simulink model "tqdtqr_rebuild_V3"  (R2021b)
settings: Solver=VariableStepAuto  StartTime=0.0  StopTime=10.0  RelTol=1e-3
undefined symbols (not defined in the file): ATQD_AfterTqMinGain_X_Deg, ATQD_APSCreepBaseTqD_X_kph, ATQD_APSCreepBaseTqD_Y_Deg, ATQD_APSCreepBaseTqR_X_kph, ATQD_APSCreepBaseTqR_Y_Deg, ATQD_APSCreepIterm_X_kph, ATQD_APSCreepIterm_Y_kph, ATQD_APSCreepPterm_X_kph, ATQD_APSCreepPterm_Y_kph, ATQD_APSDecReq_X_kph, ATQD_APSDecReq_Y_mps2, ATQD_APSDecReqCMD_X_kph, ATQD_APSDecReqTs_X_pct, ATQD_APSDecTimeGain_X_Deg, ATQD_APSDecTimeGain_Y_s, ATQD_APSReqLowSpd_X_Deg, ATQD_AutoHoldReleaseBPS_X_Deg, ATQD_AWDLoadTrqnsGain_X_kg, ATQD_AWDLoadTrqnsGain_Y_pct, ATQD_BOSEnBPSPosn_X_kph, ATQD_BOSMap_X_rpm, ATQD_BOSMap_Y_pct, ATQD_CreepBaseTqD_X_kph, ATQD_CreepBaseTqD_Y_Deg, ATQD_CreepBaseTqR_X_kph, ATQD_CreepBaseTqR_Y_Deg, ATQD_CreepBPSDisPosn_X_Deg, ATQD_CreepBPSDisPosnR_X_Deg, ATQD_CreepBPSEnPosn_X_Deg, ATQD_CreepBPSEnPosnR_X_Deg, ATQD_CreepDeltaTq_X_kph, ATQD_CreepIterm_X_kph, ATQD_CreepIterm_Y_kph, ATQD_CreepItermMaxLimit_X_pct, ATQD_CreepPreloadTime_X_kph, ATQD_CreepPreloadTq_X_kph, ATQD_CreepPreloadTq_Y_s, ATQD_CreepProtTq_X_Deg, ATQD_CreepPterm_X_kph, ATQD_CreepPterm_Y_kph, ATQD_CreepRrTqSpRat_X_rpm, ATQD_CreepRrTqSpRat_Y_Nm, ATQD_CreepTargetSpdD_X_pct, ATQD_CreepTargetSpdR_X_pct, ATQD_CreepUpLimitTq_X_rpm, ATQD_DecIneOPDHoldEnDelay_X_Deg, ATQD_DecIneOPDHoldEnDelay_Y_bar, ATQD_ECOTqMapD_X_rpm, ATQD_ECOTqMapD_Y_pct, ATQD_EMTqMapD_X_rpm, ATQD_EMTqMapD_Y_pct, ATQD_EOPDTqMapDCon_X_rpm, ATQD_EOPDTqMapDCon_Y_Deg, ATQD_EstInitVehWeight_X_c, ATQD_FAfterTqCMDGain_X_rpm, ATQD_FAfterTqCMDGain_Y_pct, ATQD_ForceLowSpd_X_Deg, ATQD_ForcePLimitSpd_X_Deg, ATQD_FrLossMAPLowV_X_rpm, ATQD_FrLossMAPLowV_Y_Nm ... (+949)
libraries: simulink x235, hcu_lib x208, tqr x63, tqd x6
(part 19 of 37)

== system tqdtqr_rebuild_V3/Input_Convert/Main function/Front//Rear ramp parameters determine/Front First order filter input tau map and determination ==
  note: Drive mode case
  note: Determine Tq by different case
  VTQD_TqTargetShaftSpd_rpm : Inport
  VTQR_EVDriveMode_enum : Inport  Port=2
  VTQD_RollRegenEnable_flg : Inport  Port=3
  VTQD_TqSourceFr_enum : Inport  Port=4
  VTQR_FEDUWhlTqReqSmoothDelay_Nm : Inport  Port=5
  VDHP_ActAPSPosn_pct : Inport  Port=6
  VINP_VehSpeed_kph : Inport  Port=7
  VTQD_LimpHomeAct_flg : Inport  Port=8
  VTQD_EVDriveModeValid_flg : Inport  Port=9
  VTQD_RegenMode_enum : Inport  Port=10
  VVMC_ACCPedalOvrd_flg : Inport  Port=11
  VVMC_CCPedalOvrd_flg : Inport  Port=12
  VTQD_PreLoadHold_flg : Inport  Port=13
  VVMC_ActMaxSlideRate_pct : Inport  Port=14
  VTQD_CreepPrLoadEnable_flg : Inport  Port=15
  VTQD_RDCActive_enum : Inport  Port=16
  VTQR_NoABSFEDUWhlTqReq_Nm : Inport  Port=17
  VTQR_RampFEDUWhlTqReq_Nm : Inport  Port=18
  VTQR_FrFirstOrderInpTq_Nm : Inport  Port=19
  VTQD_PedAccTqEn_flg : Inport  Port=20
  VTQD_PreLoadPreEn_flg : Inport  Port=21
  VVMC_MSAWhlTqActive_flg : Inport  Port=22
  VINP_FrPTCSActive_flg : Inport  Port=23
  VINP_IVISnowModeCmd_flg : Inport  Port=24
  VTQD_IVIRockModeEn_flg : Inport  Port=25
  VINP_VehicleType_enum : Inport  Port=26
  VTQD_CoordWhlTqDemFr_Nm : Inport  Port=27
  VINP_FrntAxlTrqReqDrv_Nm : Inport  Port=28
  VVMC_EstSlope_Deg : Inport  Port=29
  AND : Logic  AllPortsSameDT=off  OutDataTypeStr=boolean
  AND1 : Logic  Inputs=3  AllPortsSameDT=off  OutDataTypeStr=boolean
  AND2 : Logic  Inputs=3  AllPortsSameDT=off  OutDataTypeStr=boolean
  AND3 : Logic  AllPortsSameDT=off  OutDataTypeStr=boolean
  AND4 : Logic  AllPortsSameDT=off  OutDataTypeStr=boolean
  Abs : Abs
  Abs4 : Abs
  Add : Sum  Inputs=+-
  Add1 : Sum  Inputs=+-
  Constant : Constant  Value=ENUM_VEHICLETYPE_D31L24
  Constant1 : Constant  Value=ENUM_TQSOURCE_APS
  Constant10 : Constant  Value=KTQR_PreLoadTs_c
  Constant11 : Constant  Value=ENUM_DRIVEMODE_ECO
  Constant12 : Constant  Value=ENUM_DRIVEMODE_NRM
  Constant16 : Constant  Value=ENUM_DRIVEMODE_SPORT
  Constant2 : Constant  Value=KTQR_DriveModeCMDTqDev_Nm
  Constant3 : Constant  Value=ENUM_TQSOURCE_CC
  Constant32 : Constant  Value=KTQR_TIPOutTsAPS_pct
  Constant33 : Constant  Value=KTQR_TIPOutTsSpd_kph
  Constant34 : Constant  Value=ENUM_TQSOURCE_ADAS
  Constant5 : Constant  Value=KTQR_ARegenLatchEnTq_Nm
  Constant6 : Constant  Value=KTQR_PreLoadPreEnTs_c
  Constant7 : Constant  Value=ENUM_RDCACTSTA_NOREQUEST
  Constant8 : Constant  Value=KTQR_DriveModeChangeTq_Nm
  Constant9 : Constant  Value=ENUM_TQSOURCE_MSA
  Creep : Subsystem  TreatAsAtomicUnit=on
  Delay : Delay  DelayLength=1
  Delay1 : Delay  DelayLength=1
  Delay2 : Delay  DelayLength=1
  Detect Change : simulink/Logic and Bit Operations/Detect Change  vinit=0  OutDataTypeStr=boolean
  Drive mode : Subsystem  TreatAsAtomicUnit=on
  Equal : RelationalOperator  Operator=~=  OutDataTypeStr=boolean  RndMeth=Simplest
  Equal10 : RelationalOperator  Operator===  OutDataTypeStr=boolean  RndMeth=Simplest
  Equal11 : RelationalOperator  Operator===  OutDataTypeStr=boolean  RndMeth=Simplest
  Equal2 : RelationalOperator  Operator=~=  OutDataTypeStr=boolean  RndMeth=Simplest
  Equal9 : RelationalOperator  Operator===  OutDataTypeStr=boolean  RndMeth=Simplest
  GreaterThan2 : RelationalOperator  OutDataTypeStr=boolean  RndMeth=Simplest
  If : If  NumInputs=7  IfExpression=u1~= 0  ElseIfExpressions=u2 ~= 0, u3 ~= 0,u4~=0,u5~=0,u6~=0
  If1 : If  NumInputs=6  IfExpression=u1~= 0  ElseIfExpressions=u2 ~= 0, u3 ~= 0,u4~=0,u5~=0,u6~=0
  Less Than2 : RelationalOperator  Operator=<=  OutDataTypeStr=boolean  RndMeth=Simplest
  Logical Operator : Logic  AllPortsSameDT=off  OutDataTypeStr=boolean
  Logical Operator1 : Logic  Inputs=3  AllPortsSameDT=off  OutDataTypeStr=boolean
  Logical Operator14 : Logic  Operator=OR  Inputs=5  AllPortsSameDT=off  OutDataTypeStr=boolean
  Logical Operator2 : Logic  Operator=OR  AllPortsSameDT=off  OutDataTypeStr=boolean
  Logical Operator3 : Logic  Operator=NOT  AllPortsSameDT=off  OutDataTypeStr=boolean
  Logical Operator4 : Logic  Operator=NOT  AllPortsSameDT=off  OutDataTypeStr=boolean
  Logical Operator5 : Logic  AllPortsSameDT=off  OutDataTypeStr=boolean
  Merge : Merge  Inputs=7
  Merge1 : Merge  Inputs=7
  NOT : Logic  Operator=NOT  AllPortsSameDT=off  OutDataTypeStr=boolean
  NOT1 : Logic  Operator=NOT  AllPortsSameDT=off  OutDataTypeStr=boolean
  OR2 : Logic  Operator=OR  AllPortsSameDT=off  OutDataTypeStr=boolean
  Preleoad : Subsystem  TreatAsAtomicUnit=on
  PreleoadPreEn : Subsystem  TreatAsAtomicUnit=on
  RDCActive : Subsystem  TreatAsAtomicUnit=on
  Relational Operator : RelationalOperator  Operator=>  OutDataTypeStr=boolean  RndMeth=Simplest
  Relational Operator1 : RelationalOperator  Operator=~=  OutDataTypeStr=boolean  RndMeth=Simplest
  Relational Operator2 : RelationalOperator  Operator=<=  OutDataTypeStr=boolean  RndMeth=Simplest
  Relational Operator3 : RelationalOperator  Operator===  OutDataTypeStr=boolean  RndMeth=Simplest
  Relational Operator4 : RelationalOperator  Operator===  OutDataTypeStr=boolean  RndMeth=Simplest
  Relational Operator5 : RelationalOperator  Operator=<  OutDataTypeStr=boolean  RndMeth=Simplest
  Relational Operator6 : RelationalOperator  OutDataTypeStr=boolean  RndMeth=Simplest
  Relational Operator7 : RelationalOperator  Operator===  OutDataTypeStr=boolean  RndMeth=Simplest
  SR_Latch1 : hcu_lib/Basic_Blocks/SR_Latch
  Switch4 : Switch  Criteria=u2 > Threshold
  TIP : Subsystem  TreatAsAtomicUnit=on
  VMC : Subsystem  TreatAsAtomicUnit=on
  VTQR_ECOFEDUTs_c : tqr/TQR/Determine Torque Request/TorqueArbitrament/TorqueSmooth/Front First order filter input tau map and determination/VTQR_ECOFEDUTs_c  SystemSampleTime=-1  VariantActivationTime=update diagram  Latency=0  AutoFrameSizeCalculation=off
  VTQR_ESCAPEFEDUTs_c : tqr/TQR/Determine Torque Request/TorqueArbitrament/TorqueSmooth/Front First order filter input tau map and determination/VTQR_ESCAPEFEDUTs_c  SystemSampleTime=-1  VariantActivationTime=update diagram  Latency=0  AutoFrameSizeCalculation=off
  VTQR_LHMFEDUTs_c : tqr/TQR/Determine Torque Request/TorqueArbitrament/TorqueSmooth/Front First order filter input tau map and determination/VTQR_LHMFEDUTs_c  SystemSampleTime=-1  VariantActivationTime=update diagram  Latency=0  AutoFrameSizeCalculation=off
  VTQR_NORMALFEDUTs_c : tqr/TQR/Determine Torque Request/TorqueArbitrament/TorqueSmooth/Front First order filter input tau map and determination/VTQR_NORMALFEDUTs_c  SystemSampleTime=-1  VariantActivationTime=update diagram  Latency=0  AutoFrameSizeCalculation=off
  VTQR_SNOWFEDUTs_c : tqr/TQR/Determine Torque Request/TorqueArbitrament/TorqueSmooth/Front First order filter input tau map and determination/VTQR_SNOWFEDUTs_c  SystemSampleTime=-1  VariantActivationTime=update diagram  Latency=0  AutoFrameSizeCalculation=off
  VTQR_SPORTFEDUTs_c : tqr/TQR/Determine Torque Request/TorqueArbitrament/TorqueSmooth/Front First order filter input tau map and determination/VTQR_SPORTFEDUTs_c  SystemSampleTime=-1  VariantActivationTime=update diagram  Latency=0  AutoFrameSizeCalculation=off
  VTQR_TCSFEDUTs_c : tqr/TQR/Determine Torque Request/TorqueArbitrament/TorqueSmooth/Front First order filter input tau map and determination/VTQR_TCSFEDUTs_c  SystemSampleTime=-1  VariantActivationTime=update diagram  Latency=0  AutoFrameSizeCalculation=off
  VTQR_FrFirstOrderInpTs_c : Outport
  wires:
  VTQD_CoordWhlTqDemFr_Nm/1 -> [VTQD_CoordWhlTqDemFr_Nm]
  VINP_FrntAxlTrqReqDrv_Nm/1 -> [VINP_FrntAxlTrqReqDrv_Nm]
  VINP_VehicleType_enum/1 -> [VINP_VehicleType_enum]
  VINP_IVISnowModeCmd_flg/1 -> [VINP_IVISnowModeCmd_flg]
  VTQD_IVIRockModeEn_flg/1 -> [VTQD_IVIRockModeEn_flg]
  VINP_FrPTCSActive_flg/1 -> [VINP_FrPTCSActive_flg]
  [VTQD_PedAccTqEn_flg] -> Logical Operator14/5
  AND3/1 -> Logical Operator14/3
  Constant9/1 -> Relational Operator7/2
  [VVMC_MSAWhlTqActive_flg] -> AND3/2
  VVMC_MSAWhlTqActive_flg/1 -> [VVMC_MSAWhlTqActive_flg]
  [VTQD_TqSourceFr_enum] -> Relational Operator7/1
  Relational Operator7/1 -> AND3/1
  VTQD_PreLoadPreEn_flg/1 -> [VTQD_PreLoadPreEn_flg]
  VTQD_PedAccTqEn_flg/1 -> [VTQD_PedAccTqEn_flg]
  VVMC_ActMaxSlideRate_pct/1 -> [VVMC_ActMaxSlideRate_pct]
  VTQR_FrFirstOrderInpTq_Nm/1 -> [VTQR_FrFirstOrderInpTq_Nm]
  [VTQR_RampFEDUWhlTqReq_Nm] -> Relational Operator2/1
  Constant7/1 -> Equal2/2
  Equal2/1 -> AND/2
  [VTQD_RDCActive_enum] -> Equal2/1
  Relational Operator2/1 -> AND/1
  Constant5/1 -> Relational Operator2/2
  VTQR_RampFEDUWhlTqReq_Nm/1 -> [VTQR_RampFEDUWhlTqReq_Nm]
  VTQR_NoABSFEDUWhlTqReq_Nm/1 -> [VTQR_NoABSFEDUWhlTqReq_Nm]
  VTQD_RDCActive_enum/1 -> [VTQD_RDCActive_enum]
  VTQD_CreepPrLoadEnable_flg/1 -> [VTQD_CreepPrLoadEnable_flg]
  VTQD_PreLoadHold_flg/1 -> [VTQD_PreLoadHold_flg]
  VVMC_CCPedalOvrd_flg/1 -> [VVMC_CCPedalOvrd_flg]
  VVMC_ACCPedalOvrd_flg/1 -> [VVMC_ACCPedalOvrd_flg]
  GreaterThan2/1 -> AND2/2
  [VTQD_TqSourceFr_enum] -> Relational Operator4/1
  Relational Operator1/1 -> AND2/3
  Relational Operator3/1 -> Logical Operator14/1
  Logical Operator14/1 -> AND1/1
  Constant33/1 -> GreaterThan2/2
  Constant3/1 -> Relational Operator3/2
  Less Than2/1 -> AND2/1
  [VTQD_TqSourceFr_enum] -> Relational Operator3/1
  [VDHP_ActAPSPosn_pct] -> Less Than2/1
  Relational Operator4/1 -> Logical Operator14/2
  Constant32/1 -> Less Than2/2
  Constant34/1 -> Relational Operator4/2
  [VINP_VehSpeed_kph] -> GreaterThan2/1
  Constant1/1 -> Relational Operator1/2
  [VTQD_TqSourceFr_enum] -> Relational Operator1/1
  [VVMC_ACCPedalOvrd_flg] -> NOT/1
  [VTQD_CreepPrLoadEnable_flg] -> Logical Operator14/4
  NOT1/1 -> AND1/3
  [VVMC_CCPedalOvrd_flg] -> NOT1/1
  VTQD_RegenMode_enum/1 -> [VTQD_RegenMode_enum]
  VTQD_EVDriveModeValid_flg/1 -> [VTQD_EVDriveModeValid_flg]
  VTQD_LimpHomeAct_flg/1 -> [VTQD_LimpHomeAct_flg]
  VINP_VehSpeed_kph/1 -> [VINP_VehSpeed_kph]
  VDHP_ActAPSPosn_pct/1 -> [VDHP_ActAPSPosn_pct]
  VTQR_FEDUWhlTqReqSmoothDelay_Nm/1 -> [VTQR_FEDUWhlTqReqSmoothDelay_Nm]
  VTQD_TqSourceFr_enum/1 -> [VTQD_TqSourceFr_enum]
  VTQD_RollRegenEnable_flg/1 -> [VTQD_RollRegenEnable_flg]
  VTQR_EVDriveMode_enum/1 -> [VTQR_EVDriveMode_enum]
  VTQD_TqTargetShaftSpd_rpm/1 -> [VTQD_TqTargetShaftSpd_rpm]
  AND/1 -> [VTQR_FrRDCActiveTs_flg]  "VTQR_FrRDCActiveTs_flg"
  NOT/1 -> AND1/2
  AND1/1 -> [VTQD_ADASCreepCondition_flg]
  AND2/1 -> [VTQD_APSCondition_flg]
  [VTQR_FrRDCActiveTs_flg] -> If1/1
  If1/1 -> RDCActive/Action
  Logical Operator/1 -> If1/2
  [VTQD_ADASCreepCondition_flg] -> Logical Operator/1
  [VTQD_CreepPrLoadEnable_flg] -> Logical Operator/2
  If1/2 -> Creep/Action
  [VTQD_CreepPrLoadEnable_flg] -> Logical Operator4/1
  Logical Operator4/1 -> Logical Operator5/2
  [VTQD_ADASCreepCondition_flg] -> Logical Operator5/1
  Logical Operator5/1 -> If1/3
  If1/3 -> VMC/Action
  [VTQD_APSCondition_flg] -> If1/4
  If1/4 -> TIP/Action
  [VTQD_PreLoadHold_flg] -> If1/5
  If1/5 -> Preleoad/Action
  Constant10/1 -> Preleoad/1(KTQR_PreLoadTs_c)
  RDCActive/1(VTQR_RDCActiveFEDUTs_c) -> [VTQR_RDCActiveFEDUTs_c]
  Creep/1(VTQR_CreepFEDUTs_c) -> [VTQR_CreepFEDUTs_c]
  VMC/1(VTQR_VMCFEDUTs_c) -> [VTQR_VMCFEDUTs_c]
  TIP/1(VTQR_FEDUTIPOutTs_c) -> [VTQR_FEDUTIPOutTs_c]
  Preleoad/1(VTQR_PreLoadTs_c) -> [VTQR_PreLoadTs_c]
  Merge1/1 -> VTQR_FrFirstOrderInpTs_c/1  "VTQR_FrFirstOrderInpTs_c"
  [VTQD_RegenMode_enum] -> RDCActive/1(VTQD_RegenMode_enum)
  [VVMC_ActMaxSlideRate_pct] -> RDCActive/2(VVMC_ActMaxSlideRate_pct)
  [VTQR_FEDUWhlTqReqSmoothDelay_Nm] -> Creep/1(VTQR_FEDUWhlTqReqSmoothDelay_Nm)
  [VTQD_TqTargetShaftSpd_rpm] -> Creep/2(VTQD_TqTargetShaftSpd_rpm)
  [VTQR_FEDUWhlTqReqSmoothDelay_Nm] -> VMC/1(VTQR_FEDUWhlTqReqSmoothDelay_Nm)
  [VTQD_TqTargetShaftSpd_rpm] -> VMC/2(VTQD_TqTargetShaftSpd_rpm)
  [VTQD_TqTargetShaftSpd_rpm] -> TIP/1(VTQD_TqTargetShaftSpd_rpm)
  [VTQD_PreLoadPreEn_flg] -> If1/6
  ? -> ?
  ? -> ?
  Constant6/1 -> PreleoadPreEn/1(KTQR_PreLoadPreEnTs_c)
  PreleoadPreEn/1(VTQR_PreLoadPreEnTs_c) -> [VTQR_PreLoadPreEnTs_c]
  [VTQR_RDCActiveFEDUTs_c] -> Merge1/1
  [VTQR_CreepFEDUTs_c] -> Merge1/2
  [VTQR_VMCFEDUTs_c] -> Merge1/3
  [VTQR_FEDUTIPOutTs_c] -> Merge1/4
  [VTQR_PreLoadTs_c] -> Merge1/5
  [VTQR_PreLoadPreEnTs_c] -> Merge1/6
  Logical Operator1/1 -> If/2
  Relational Operator/1 -> Logical Operator1/3
  [VINP_FrntAxlTrqReqDrv_Nm] -> Relational Operator/2
  [VTQR_FEDUWhlTqReqSmoothDelay_Nm] -> VTQR_LHMFEDUTs_c/1
  VTQR_ESCAPEFEDUTs_c/1 -> [VTQR_ESCAPEFEDUTs_c]  "VTQR_ESCAPEFEDUTs_c"
  VTQR_SPORTFEDUTs_c/1 -> [VTQR_SPORTFEDUTs_c]  "VTQR_SPORTFEDUTs_c"
  Equal/1 -> Logical Operator1/2
  [VINP_VehicleType_enum] -> Equal/1
  VTQR_TCSFEDUTs_c/1 -> [VTQR_TCSFEDUTs_c]  "VTQR_TCSFEDUTs_c"
  [VTQR_FEDUWhlTqReqSmoothDelay_Nm] -> VTQR_NORMALFEDUTs_c/1
  [VTQR_FEDUWhlTqReqSmoothDelay_Nm] -> VTQR_TCSFEDUTs_c/1
  VTQR_LHMFEDUTs_c/1 -> [VTQR_LHMFEDUTs_c]  "VTQR_LHMFEDUTs_c"
  [VTQR_FEDUWhlTqReqSmoothDelay_Nm] -> VTQR_SNOWFEDUTs_c/1
  VTQR_NORMALFEDUTs_c/1 -> [VTQR_NORMALFEDUTs_c]  "VTQR_NORMALFEDUTs_c"
  [VTQD_TqTargetShaftSpd_rpm] -> VTQR_NORMALFEDUTs_c/2
  If/6 -> VTQR_ECOFEDUTs_c/Action
  [VINP_IVISnowModeCmd_flg] -> If/4
  If/3 -> VTQR_ESCAPEFEDUTs_c/Action
  If/7 -> VTQR_SPORTFEDUTs_c/Action
  [VTQD_TqTargetShaftSpd_rpm] -> VTQR_ESCAPEFEDUTs_c/2
  Equal11/1 -> If/5
  [VTQR_FEDUWhlTqReqSmoothDelay_Nm] -> VTQR_ECOFEDUTs_c/1
  [VTQD_IVIRockModeEn_flg] -> If/3
  Equal9/1 -> If/7
  Equal10/1 -> If/6
  If/2 -> VTQR_TCSFEDUTs_c/Action
  [VINP_FrPTCSActive_flg] -> Logical Operator1/1
  [VTQD_TqTargetShaftSpd_rpm] -> VTQR_TCSFEDUTs_c/2
  If/4 -> VTQR_SNOWFEDUTs_c/Action
  [VTQD_RegenMode_enum] -> VTQR_NORMALFEDUTs_c/3
  VTQR_ECOFEDUTs_c/1 -> [VTQR_ECOFEDUTs_c]  "VTQR_ECOFEDUTs_c"
  VTQR_SNOWFEDUTs_c/1 -> [VTQR_SNOWFEDUTs_c]  "VTQR_SNOWFEDUTs_c"
  [VTQD_TqTargetShaftSpd_rpm] -> VTQR_ECOFEDUTs_c/2
  If/1 -> VTQR_LHMFEDUTs_c/Action
  [VTQD_CoordWhlTqDemFr_Nm] -> Relational Operator/1
  [VTQD_RollRegenEnable_flg] -> VTQR_ECOFEDUTs_c/4
  [VTQR_FEDUWhlTqReqSmoothDelay_Nm] -> VTQR_ESCAPEFEDUTs_c/1
  [VTQD_RegenMode_enum] -> VTQR_ECOFEDUTs_c/3
  [VTQD_TqTargetShaftSpd_rpm] -> VTQR_SNOWFEDUTs_c/2
  [VTQD_LimpHomeAct_flg] -> Logical Operator2/1
  [VTQD_RegenMode_enum] -> VTQR_SPORTFEDUTs_c/3
  Logical Operator2/1 -> If/1
  [VTQR_FEDUWhlTqReqSmoothDelay_Nm] -> VTQR_SPORTFEDUTs_c/1
  Constant/1 -> Equal/2
  Constant11/1 -> Equal10/2
  If/5 -> VTQR_NORMALFEDUTs_c/Action
  [VTQD_TqTargetShaftSpd_rpm] -> VTQR_LHMFEDUTs_c/2
  [VTQR_EVDriveMode_enum] -> Equal9/1
  [VTQD_TqTargetShaftSpd_rpm] -> VTQR_SPORTFEDUTs_c/2
  Logical Operator3/1 -> Logical Operator2/2
  Constant12/1 -> Equal11/2
  [VTQR_EVDriveMode_enum] -> Equal10/1
  [VTQR_EVDriveMode_enum] -> Equal11/1
  [VTQD_EVDriveModeValid_flg] -> Logical Operator3/1
  Constant16/1 -> Equal9/2
  [VTQR_EVDriveMode_enum] -> Detect Change/1
  [VTQR_FrFirstOrderInpTq_Nm] -> Delay1/1
  [VTQR_ESCAPEFEDUTs_c] -> Merge/3
  [VTQR_ECOFEDUTs_c] -> Merge/6
  [VTQR_SPORTFEDUTs_c] -> Merge/7
  [VTQR_FrFirstOrderInpTq_Nm] -> Add/2
  [VTQR_LHMFEDUTs_c] -> Merge/1
  Delay/1 -> Switch4/1
  [VTQR_TCSFEDUTs_c] -> Merge/2
  Delay1/1 -> Add1/1
  Add/1 -> Abs/1
  Abs/1 -> Relational Operator5/1
  Add1/1 -> Abs4/1
  Detect Change/1 -> SR_Latch1/1
  Switch4/1 -> [VTQR_FEDUTs_c], Delay/1  "VTQR_FEDUTs_c"
  Abs4/1 -> Relational Operator6/1
  [VTQR_FrDrModChangeReset_flg] -> SR_Latch1/2
  Constant8/1 -> Relational Operator5/2
  [VTQR_FrFirstOrderInpTq_Nm] -> Add1/2
  SR_Latch1/1 -> Switch4/2, [VTQR_FrDrModTsLatch_flg]  "VTQR_FrDrModLatch_flg"
  Relational Operator6/1 -> AND4/1
  [VTQR_FrDrModTsLatch_flg] -> Delay2/1
  [VTQR_SNOWFEDUTs_c] -> Merge/4
  Relational Operator5/1 -> OR2/1
  OR2/1 -> [VTQR_FrDrModChangeReset_flg]  "VTQR_FrDrModChangeReset_flg"
  Constant2/1 -> Relational Operator6/2
  [VTQR_NoABSFEDUWhlTqReq_Nm] -> Add/1
  AND4/1 -> OR2/2
  Merge/1 -> Switch4/3
  Delay2/1 -> AND4/2
  [VTQR_NORMALFEDUTs_c] -> Merge/5
  If1/6 -> PreleoadPreEn/Action
  If1/7 -> Drive mode/Action
  [VTQR_FEDUTs_c] -> Drive mode/1(VTQR_FEDUTs_c)
  Drive mode/1(VTQR_OutFEDUTs_c) -> [VTQR_OutFEDUTs_c]
  [VTQR_OutFEDUTs_c] -> Merge1/7
  VVMC_EstSlope_Deg/1 -> [VVMC_EstSlope_Deg]
  [VVMC_EstSlope_Deg] -> Creep/3(VVMC_EstSlope_Deg)

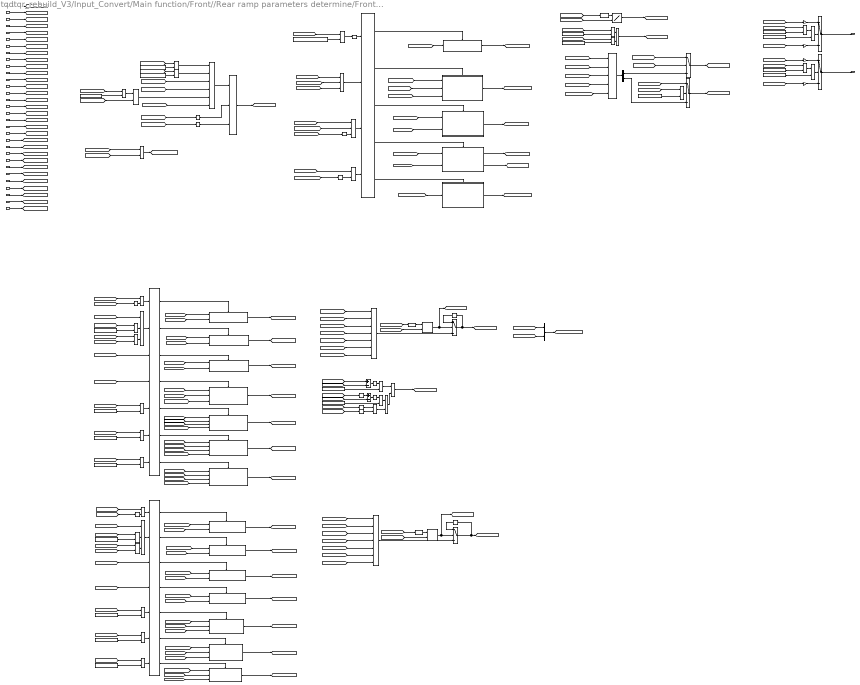
== system tqdtqr_rebuild_V3/Input_Convert/Main function/Front//Rear ramp parameters determine/Front wheel rate limit determination ==
  note: Drive mode case
  note: Merge result and decide final torque
  note: Determin torque by different cases
  note: Check direction
  VTQR_FrTqZeroTrans_enum : Inport
  VTQD_TqSourceFr_enum : Inport  Port=2
  VTQD_TqTargetShaftSpd_rpm : Inport  Port=3
  VTQD_LimpHomeAct_flg : Inport  Port=4
  VTQR_EVDriveMode_enum : Inport  Port=5
  VDHP_ActAPSPosn_pct : Inport  Port=6
  VTQR_FEDUWhlTqReqSmoothDelay_Nm : Inport  Port=7
  VTQD_EVDriveModeValid_flg : Inport  Port=8
  VTQD_RegenMode_enum : Inport  Port=9
  VVMC_ACCPedalOvrd_flg : Inport  Port=10
  VVMC_CCPedalOvrd_flg : Inport  Port=11
  VTQD_CreepPrLoadEnable_flg : Inport  Port=12
  VTQD_RegenTqLimitEn_flg : Inport  Port=13
  VTQD_RDCActive_enum : Inport  Port=14
  VTQD_PreLoadPreEn_flg : Inport  Port=15
  VTQR_NoABSFEDUWhlTqReq_Nm : Inport  Port=16
  VTQR_RampFEDUWhlTqReq_Nm : Inport  Port=17
  VTQR_FrFirstOrderInpTq_Nm : Inport  Port=18
  VVMC_ActMaxSlideRate_pct : Inport  Port=19
  VTQD_PedAccTqEn_flg : Inport  Port=20
  VVMC_MSAWhlTqActive_flg : Inport  Port=21
  VINP_FrPTCSActive_flg : Inport  Port=22
  VTQD_GearActualPosn_enum : Inport  Port=23
  VINP_IVISnowModeCmd_flg : Inport  Port=24
  VTQD_IVIRockModeEn_flg : Inport  Port=25
  VTQD_FrShaftSpd_rpm : Inport  Port=26
  VINP_VehicleType_enum : Inport  Port=27
  VTQD_CoordWhlTqDemFr_Nm : Inport  Port=28
  VINP_FrntAxlTrqReqDrv_Nm : Inport  Port=29
  VTQD_FrZeroPointIncDec_Nm : Inport  Port=30
  VVMC_EstSlope_Deg : Inport  Port=31
  AND{,2,4..6,8} (6 alike) : Logic  AllPortsSameDT=off  OutDataTypeStr=boolean
  AND7 : Logic  Inputs=3  AllPortsSameDT=off  OutDataTypeStr=boolean
  Abs : Abs
  Abs4 : Abs
  Add : Sum  Inputs=+-
  Add1 : Sum  Inputs=+-
  Constant : Constant  Value=ENUM_VEHICLETYPE_D31L24
  Constant10 : Constant  Value=ENUM_TQSOURCE_MSA
  Constant11 : Constant  Value=KTQR_DriveModeCMDTqDev_Nm
  Constant12 : Constant  Value=KTQR_ARegenLatchEnTq_Nm
  Constant13 : Constant  Value=ENUM_TQSOURCE_CC
  Constant14 : Constant  Value=ENUM_DRIVEMODE_ECO
  Constant15 : Constant  Value=ENUM_DRIVEMODE_NRM
  Constant17 : Constant  Value=ENUM_DRIVEMODE_SPORT
  Constant18 : Constant  Value=ENUM_GEARACTUALPOSN_R
  Constant19 : Constant  Value=KTQR_NewRampArchSW_flg
  Constant2 : Constant  Value=ENUM_RDCACTSTA_NOREQUEST
  Constant20 : Constant  Value=ENUM_GEARACTUALPOSN_R
  Constant21 : Constant  Value=KTQR_NewRampArchSW_flg
  Constant22 : Constant  Value=ENUM_VEHICLETYPE_D31L24
  Constant23 : Constant  Value=ENUM_TQSOURCE_ADAS
  Constant4 : Constant  Value=ENUM_TQZEROTRANS_NOZEROTRANS
  Constant5 : Constant  Value=KTQR_DriveModeChangeTq_Nm
  Constant6 : Constant  Value=KTQR_RegenTqLimitDecSW_flg
  Constant7 : Constant  Value=ENUM_DRIVEMODE_ECO
  Constant8 : Constant  Value=ENUM_DRIVEMODE_NRM
  Constant9 : Constant  Value=ENUM_DRIVEMODE_SPORT
  Data Type Conversion : DataTypeConversion  OutDataTypeStr=single
  Delay{,1..4} (5 alike) : Delay  DelayLength=1
  Demux : Demux  Outputs=2
  Detect Change : simulink/Logic and Bit Operations/Detect Change  vinit=0  OutDataTypeStr=boolean
  Detect Change1 : simulink/Logic and Bit Operations/Detect Change  vinit=0  OutDataTypeStr=boolean
  Drive mode : Subsystem  TreatAsAtomicUnit=on
  Equal{,1,5..6,8,12..13,15} (8 alike) : RelationalOperator  Operator===  OutDataTypeStr=boolean  RndMeth=Simplest
  Equal2 : RelationalOperator  Operator=~=  OutDataTypeStr=boolean  RndMeth=Simplest
  Equal3 : RelationalOperator  Operator=~=  OutDataTypeStr=boolean  RndMeth=Simplest
  Equal4 : RelationalOperator  Operator=~=  OutDataTypeStr=boolean  RndMeth=Simplest
  Gain : Gain
  Gain2 : Gain  Gain=-1
  Gain3 : Gain
  Gain4 : Gain  Gain=-1
  If1 : If  NumInputs=7  IfExpression=u1~= 0  ElseIfExpressions=u2 ~= 0, u3 ~= 0,u4 ~= 0,u5~=0, u6~=0, u7~=0  ShowElse=off
  If2 : If  NumInputs=7  IfExpression=u1~= 0  ElseIfExpressions=u2 ~= 0, u3 ~= 0,u4 ~= 0, u5~=0, u6~=0, u7~=0  ShowElse=off
  If3 : If  NumInputs=4  IfExpression=u1~= 0  ElseIfExpressions=u2 ~= 0, u3 ~= 0,u4~=0
  Logical Operator{,2..3,10} (4 alike) : Logic  Inputs=3  AllPortsSameDT=off  OutDataTypeStr=boolean
  Logical Operator{1,5,8,11,13} (5 alike) : Logic  Operator=NOT  AllPortsSameDT=off  OutDataTypeStr=boolean
  Logical Operator12 : Logic  AllPortsSameDT=off  OutDataTypeStr=boolean
  Logical Operator4 : Logic  Operator=OR  AllPortsSameDT=off  OutDataTypeStr=boolean
  Logical Operator6 : Logic  Operator=OR  AllPortsSameDT=off  OutDataTypeStr=boolean
  Logical Operator9 : Logic  Operator=OR  Inputs=6  AllPortsSameDT=off  OutDataTypeStr=boolean
  MTQR_AltRDCActiveFEDUInc_Z_Nm : Lookup_n-D  BreakpointsForDimension1=ATQR_AltRDCActiveFEDUInc_Y_enum  BreakpointsForDimension2=ATQR_AltRDCActiveFEDUInc_X_pct  Table=MTQR_AltRDCActiveFEDUInc_Z_Nm  TableDataTypeStr=Inherit: Inherit from 'Table data'  ExtrapMethod=Clip  InternalRulePriority=Speed  RndMeth=Simplest  InputSameDT=on
      settings: InputPortMap=u0,u1
  Merge : Merge  Inputs=5
  Merge1 : Merge  Inputs=7
  Merge2 : Merge  Inputs=7
  Mux : Mux  Inputs=2
  NOT2 : Logic  Operator=NOT  AllPortsSameDT=off  OutDataTypeStr=boolean
  NOT3 : Logic  Operator=NOT  AllPortsSameDT=off  OutDataTypeStr=boolean
  OR1 : Logic  Operator=OR  AllPortsSameDT=off  OutDataTypeStr=boolean
  OR2 : Logic  Operator=OR  AllPortsSameDT=off  OutDataTypeStr=boolean
  OR3 : Logic  Operator=OR  AllPortsSameDT=off  OutDataTypeStr=boolean
  Relational Operator{1,10..12} (4 alike) : RelationalOperator  Operator===  OutDataTypeStr=boolean  RndMeth=Simplest
  Relational Operator2 : RelationalOperator  Operator=<=  OutDataTypeStr=boolean  RndMeth=Simplest
  Relational Operator5 : RelationalOperator  Operator=<  OutDataTypeStr=boolean  RndMeth=Simplest
  Relational Operator6 : RelationalOperator  OutDataTypeStr=boolean  RndMeth=Simplest
  Relational Operator8 : RelationalOperator  Operator=>  OutDataTypeStr=boolean  RndMeth=Simplest
  Relational Operator9 : RelationalOperator  Operator=>  OutDataTypeStr=boolean  RndMeth=Simplest
  SR_Latch1 : hcu_lib/Basic_Blocks/SR_Latch
  SR_Latch2 : hcu_lib/Basic_Blocks/SR_Latch
  Switch{,7..9} (4 alike) : Switch  Criteria=u2 ~= 0
      settings: AttributesFormatString=%<Criteria>
  Switch4 : Switch  Criteria=u2 > Threshold
  Switch5 : Switch  Criteria=u2 > Threshold
  VTQD_OutFrZeroPointIncDec_Nm : Subsystem  TreatAsAtomicUnit=on
  VTQR_CreepFEDUTqIncDecSR_Nm : Subsystem  TreatAsAtomicUnit=on
  VTQR_ECOFEDURateLimitDec_Nm : tqr/TQR/Determine Torque Request/TorqueArbitrament/TorqueSmooth/Front wheel rate limit determination/VTQR_ECOFEDURateLimitDec_Nm  SystemSampleTime=-1  VariantActivationTime=update diagram  Latency=0  AutoFrameSizeCalculation=off
  VTQR_ECOFEDURateLimitInc_Nm : tqr/TQR/Determine Torque Request/TorqueArbitrament/TorqueSmooth/Front wheel rate limit determination/VTQR_ECOFEDURateLimitInc_Nm  SystemSampleTime=-1  VariantActivationTime=update diagram  Latency=0  AutoFrameSizeCalculation=off
  VTQR_ESCAPEFEDURateLimitDec_Nm : tqr/TQR/Determine Torque Request/TorqueArbitrament/TorqueSmooth/Front wheel rate limit determination/VTQR_ESCAPEFEDURateLimitDec_Nm  SystemSampleTime=-1  VariantActivationTime=update diagram  Latency=0  AutoFrameSizeCalculation=off
  VTQR_ESCAPEFEDURateLimitInc_Nm : tqr/TQR/Determine Torque Request/TorqueArbitrament/TorqueSmooth/Front wheel rate limit determination/VTQR_ESCAPEFEDURateLimitInc_Nm  SystemSampleTime=-1  VariantActivationTime=update diagram  Latency=0  AutoFrameSizeCalculation=off
  VTQR_FrPreLoadTqIncDec_Nm : Subsystem  TreatAsAtomicUnit=on
  VTQR_LHMFEDURateLimitDec_Nm : tqr/TQR/Determine Torque Request/TorqueArbitrament/TorqueSmooth/Front wheel rate limit determination/VTQR_LHMFEDURateLimitDec_Nm  SystemSampleTime=-1  VariantActivationTime=update diagram  Latency=0  AutoFrameSizeCalculation=off
  VTQR_LHMFEDURateLimitInc_Nm : tqr/TQR/Determine Torque Request/TorqueArbitrament/TorqueSmooth/Front wheel rate limit determination/VTQR_LHMFEDURateLimitInc_Nm  SystemSampleTime=-1  VariantActivationTime=update diagram  Latency=0  AutoFrameSizeCalculation=off
  VTQR_NORMALFEDURateLimitDec_Nm : tqr/TQR/Determine Torque Request/TorqueArbitrament/TorqueSmooth/Front wheel rate limit determination/VTQR_NORMALFEDURateLimitDec_Nm  SystemSampleTime=-1  VariantActivationTime=update diagram  Latency=0  AutoFrameSizeCalculation=off
  VTQR_NORMALFEDURateLimitInc_Nm : tqr/TQR/Determine Torque Request/TorqueArbitrament/TorqueSmooth/Front wheel rate limit determination/VTQR_NORMALFEDURateLimitInc_Nm  SystemSampleTime=-1  VariantActivationTime=update diagram  Latency=0  AutoFrameSizeCalculation=off
  VTQR_SNOWFEDURateLimitDec_Nm : tqr/TQR/Determine Torque Request/TorqueArbitrament/TorqueSmooth/Front wheel rate limit determination/VTQR_SNOWFEDURateLimitDec_Nm  SystemSampleTime=-1  VariantActivationTime=update diagram  Latency=0  AutoFrameSizeCalculation=off
  VTQR_SNOWFEDURateLimitInc_Nm : tqr/TQR/Determine Torque Request/TorqueArbitrament/TorqueSmooth/Front wheel rate limit determination/VTQR_SNOWFEDURateLimitInc_Nm  SystemSampleTime=-1  VariantActivationTime=update diagram  Latency=0  AutoFrameSizeCalculation=off
  VTQR_SPORTFEDURateLimitDec_Nm : tqr/TQR/Determine Torque Request/TorqueArbitrament/TorqueSmooth/Front wheel rate limit determination/VTQR_SPORTFEDURateLimitDec_Nm  SystemSampleTime=-1  VariantActivationTime=update diagram  Latency=0  AutoFrameSizeCalculation=off
  VTQR_SPORTFEDURateLimitInc_Nm : tqr/TQR/Determine Torque Request/TorqueArbitrament/TorqueSmooth/Front wheel rate limit determination/VTQR_SPORTFEDURateLimitInc_Nm  SystemSampleTime=-1  VariantActivationTime=update diagram  Latency=0  AutoFrameSizeCalculation=off
  VTQR_TCSFEDURateLimitDec_Nm : tqr/TQR/Determine Torque Request/TorqueArbitrament/TorqueSmooth/Front wheel rate limit determination/VTQR_TCSFEDURateLimitDec_Nm  SystemSampleTime=-1  VariantActivationTime=update diagram  Latency=0  AutoFrameSizeCalculation=off
  VTQR_TCSFEDURateLimitInc_Nm : tqr/TQR/Determine Torque Request/TorqueArbitrament/TorqueSmooth/Front wheel rate limit determination/VTQR_TCSFEDURateLimitInc_Nm  SystemSampleTime=-1  VariantActivationTime=update diagram  Latency=0  AutoFrameSizeCalculation=off
  VTQR_VMCFEDUIncDec_Nm : Subsystem  TreatAsAtomicUnit=on
  VTQR_FrRateLimitInc_Nm : Outport
  VTQR_FrRateLimitDec_Nm : Outport  Port=2
  wires:
  VTQD_CoordWhlTqDemFr_Nm/1 -> [VTQD_CoordWhlTqDemFr_Nm]
  VINP_FrntAxlTrqReqDrv_Nm/1 -> [VINP_FrntAxlTrqReqDrv_Nm]
  VINP_VehicleType_enum/1 -> [VINP_VehicleType_enum]
  VTQD_FrShaftSpd_rpm/1 -> [VTQD_FrShaftSpd_rpm]
  VINP_IVISnowModeCmd_flg/1 -> [VINP_IVISnowModeCmd_flg]
  VTQD_IVIRockModeEn_flg/1 -> [VTQD_IVIRockModeEn_flg]
  Switch9/1 -> VTQR_FrRateLimitDec_Nm/1  "VTQR_FrRateLimitDec_Nm"
  [VTQR_OrigFrRateLimitDec_Nm] -> Gain3/1
  [VTQR_OrigFrRateLimitInc_Nm] -> Gain/1
  [VTQD_GearActualPosn_enum] -> Equal1/1
  Constant20/1 -> Equal1/2
  Gain3/1 -> Switch9/3
  AND6/1 -> Switch9/2
  Equal1/1 -> AND6/1
  Constant21/1 -> AND6/2
  [VTQR_OrigFrRateLimitInc_Nm] -> Gain4/1
  Gain4/1 -> Switch9/1
  Gain2/1 -> Switch8/1
  [VTQR_OrigFrRateLimitDec_Nm] -> Gain2/1
  Constant19/1 -> AND5/2
  Equal/1 -> AND5/1
  AND5/1 -> Switch8/2
  Switch7/1 -> [VTQR_OrigFrRateLimitDec_Nm]  "VTQR_OrigFrRateLimitDec_Nm"
  Gain/1 -> Switch8/3
  Switch/1 -> [VTQR_OrigFrRateLimitInc_Nm]  "VTQR_OrigFrRateLimitInc_Nm"
  Switch8/1 -> VTQR_FrRateLimitInc_Nm/1  "VTQR_FrRateLimitInc_Nm"
  Constant18/1 -> Equal/2
  [VTQD_GearActualPosn_enum] -> Equal/1
  VTQD_GearActualPosn_enum/1 -> [VTQD_GearActualPosn_enum]
  VINP_FrPTCSActive_flg/1 -> [VINP_FrPTCSActive_flg]
  VTQD_PedAccTqEn_flg/1 -> [VTQD_PedAccTqEn_flg]
  VVMC_MSAWhlTqActive_flg/1 -> [VVMC_MSAWhlTqActive_flg]
  Constant6/1 -> AND2/2
  [VTQD_RegenTqLimitEn_flg] -> AND2/1
  AND2/1 -> Switch7/2
  [VTQR_VMCFEDUTqDecSR_Nm] -> Switch7/1
  Demux/2 -> Switch7/3
  VVMC_ActMaxSlideRate_pct/1 -> [VVMC_ActMaxSlideRate_pct]
  VTQD_RegenTqLimitEn_flg/1 -> [VTQD_RegenTqLimitEn_flg]
  [VTQR_RDCActiveFEDUInc_Nm] -> Switch/1
  Data Type Conversion/1 -> MTQR_AltRDCActiveFEDUInc_Z_Nm/1
  [VVMC_ActMaxSlideRate_pct] -> MTQR_AltRDCActiveFEDUInc_Z_Nm/2
  MTQR_AltRDCActiveFEDUInc_Z_Nm/1 -> [VTQR_RDCActiveFEDUInc_Nm]  "VTQR_RDCActiveFEDUInc_Nm"
  [VTQD_RegenMode_enum] -> Data Type Conversion/1
  VTQR_FrFirstOrderInpTq_Nm/1 -> [VTQR_FrFirstOrderInpTq_Nm]
  AND/1 -> [VTQR_FrRDCActRateLimitInc_flg]  "VTQR_FrRDCActRateLimitInc_flg"
  Constant12/1 -> Relational Operator2/2
  [VTQR_RampFEDUWhlTqReq_Nm] -> Relational Operator2/1
  Equal2/1 -> AND/2
  Constant2/1 -> Equal2/2
  [VTQD_RDCActive_enum] -> Equal2/1
  Relational Operator2/1 -> AND/1
  VTQR_RampFEDUWhlTqReq_Nm/1 -> [VTQR_RampFEDUWhlTqReq_Nm]
  VTQR_NoABSFEDUWhlTqReq_Nm/1 -> [VTQR_NoABSFEDUWhlTqReq_Nm]
  VTQD_RDCActive_enum/1 -> [VTQD_RDCActive_enum]
  VTQD_PreLoadPreEn_flg/1 -> [VTQD_PreLoadPreEn_flg]
  VTQD_CreepPrLoadEnable_flg/1 -> [VTQD_CreepPrLoadEnable_flg]
  Demux/1 -> Switch/3
  [VTQR_FrRDCActRateLimitInc_flg] -> Switch/2
  VVMC_CCPedalOvrd_flg/1 -> [VVMC_CCPedalOvrd_flg]
  VVMC_ACCPedalOvrd_flg/1 -> [VVMC_ACCPedalOvrd_flg]
  VTQD_RegenMode_enum/1 -> [VTQD_RegenMode_enum]
  VTQD_EVDriveModeValid_flg/1 -> [VTQD_EVDriveModeValid_flg]
  VTQR_FEDUWhlTqReqSmoothDelay_Nm/1 -> [VTQR_FEDUWhlTqReqSmoothDelay_Nm]
  VDHP_ActAPSPosn_pct/1 -> [VDHP_ActAPSPosn_pct]
  VTQR_EVDriveMode_enum/1 -> [VTQR_EVDriveMode_enum]
  VTQD_LimpHomeAct_flg/1 -> [VTQD_LimpHomeAct_flg]
  VTQD_TqTargetShaftSpd_rpm/1 -> [VTQD_TqTargetShaftSpd_rpm]
  VTQD_TqSourceFr_enum/1 -> [VTQD_TqSourceFr_enum]
  VTQR_FrTqZeroTrans_enum/1 -> [VTQR_FrTqZeroTrans_enum]
  VTQD_FrZeroPointIncDec_Nm/1 -> [VTQD_FrZeroPointIncDec_Nm]
  Constant4/1 -> Relational Operator1/2
  Logical Operator8/1 -> If3/1
  Relational Operator1/1 -> Logical Operator8/1
  [VTQR_FrTqZeroTrans_enum] -> Relational Operator1/1
  If3/1 -> VTQD_OutFrZeroPointIncDec_Nm/Action
  [VTQD_FrZeroPointIncDec_Nm] -> VTQD_OutFrZeroPointIncDec_Nm/1(VTQD_FrZeroPointIncDec_Nm)
  Constant10/1 -> Relational Operator12/2
  [VVMC_ACCPedalOvrd_flg] -> NOT2/1
  [VTQD_PedAccTqEn_flg] -> Logical Operator9/6
  Logical Operator9/1 -> AND7/1
  [VTQD_TqSourceFr_enum] -> Relational Operator11/1
  [VTQD_TqSourceFr_enum] -> Relational Operator10/1
  Relational Operator11/1 -> Logical Operator9/2
  [VVMC_MSAWhlTqActive_flg] -> AND8/2
  [VVMC_CCPedalOvrd_flg] -> NOT3/1
  NOT3/1 -> AND7/3
  Constant13/1 -> Relational Operator10/2
  Relational Operator12/1 -> AND8/1
  Constant23/1 -> Relational Operator11/2
  [VTQD_PreLoadPreEn_flg] -> Logical Operator9/4
  [VTQD_TqSourceFr_enum] -> Relational Operator12/1
  [VTQD_CreepPrLoadEnable_flg] -> Logical Operator9/3
  Relational Operator10/1 -> Logical Operator9/1
  AND8/1 -> Logical Operator9/5
  NOT2/1 -> AND7/2
  AND7/1 -> [VTQR_ADASCase_flg]
  [VTQD_PreLoadPreEn_flg] -> OR1/2
  OR1/1 -> [VTQR_PreLoadCase_flg]
  [VTQD_CreepPrLoadEnable_flg] -> OR1/1
  [VTQR_ADASCase_flg] -> Logical Operator/1
  [VTQR_PreLoadCase_flg] -> Logical Operator/2
  [VTQD_CreepPrLoadEnable_flg] -> Logical Operator/3
  Logical Operator/1 -> If3/2
  If3/2 -> VTQR_CreepFEDUTqIncDecSR_Nm/Action
  [VTQR_FEDUWhlTqReqSmoothDelay_Nm] -> VTQR_CreepFEDUTqIncDecSR_Nm/1(VTQR_FEDUWhlTqReqSmoothDelay_Nm)
  [VTQD_TqTargetShaftSpd_rpm] -> VTQR_CreepFEDUTqIncDecSR_Nm/2(VTQD_TqTargetShaftSpd_rpm)
  [VTQR_PreLoadCase_flg] -> Logical Operator10/2
  [VTQR_ADASCase_flg] -> Logical Operator10/1
  Logical Operator10/1 -> If3/3
  Logical Operator11/1 -> Logical Operator10/3
  [VTQD_CreepPrLoadEnable_flg] -> Logical Operator11/1
  [VTQR_FEDUWhlTqReqSmoothDelay_Nm] -> VTQR_FrPreLoadTqIncDec_Nm/1(VTQR_FEDUWhlTqReqSmoothDelay_Nm)
  [VTQD_TqTargetShaftSpd_rpm] -> VTQR_FrPreLoadTqIncDec_Nm/2(VTQD_TqTargetShaftSpd_rpm)
  If3/3 -> VTQR_FrPreLoadTqIncDec_Nm/Action
  [VTQR_ADASCase_flg] -> Logical Operator12/1
  [VTQR_PreLoadCase_flg] -> Logical Operator13/1
  Logical Operator12/1 -> If3/4
  Logical Operator13/1 -> Logical Operator12/2
  [VTQR_FEDUWhlTqReqSmoothDelay_Nm] -> VTQR_VMCFEDUIncDec_Nm/1(VTQR_FEDUWhlTqReqSmoothDelay_Nm)
  [VTQD_TqTargetShaftSpd_rpm] -> VTQR_VMCFEDUIncDec_Nm/2(VTQD_TqTargetShaftSpd_rpm)
  VTQD_OutFrZeroPointIncDec_Nm/1(VTQD_OutFrZeroPointIncDec_Nm) -> [VTQD_OutFrZeroPointIncDec_Nm]  "VTQD_OutFrZeroPointIncDec_Nm"
  VTQR_CreepFEDUTqIncDecSR_Nm/1(VTQR_CreepFEDUTqIncDecSR_Nm) -> [VTQR_CreepFEDUTqIncDecSR_Nm]  "VTQR_CreepFEDUTqIncDecSR_Nm"
  VTQR_FrPreLoadTqIncDec_Nm/1(VTQR_FrPreLoadTqIncDec_Nm) -> [VTQR_FrPreLoadTqIncDec_Nm]  "VTQR_FrPreLoadTqIncDec_Nm"
  VTQR_VMCFEDUIncDec_Nm/1(VTQR_VMCFEDUIncDec_Nm) -> [VTQR_VMCFEDUIncDec_Nm]  "VTQR_VMCFEDUIncDec_Nm"
  [VTQD_OutFrZeroPointIncDec_Nm] -> Merge/1
  [VTQR_CreepFEDUTqIncDecSR_Nm] -> Merge/2
  [VTQR_FrPreLoadTqIncDec_Nm] -> Merge/3
  [VTQR_VMCFEDUIncDec_Nm] -> Merge/4
  Merge/1 -> Demux/1
  VTQR_VMCFEDUIncDec_Nm/2(VTQR_VMCFEDUIncDec_Nm1) -> [VTQR_VMCFEDUTqDecSR_Nm]
  [VTQR_EVDriveMode_enum] -> Equal8/1
  [VTQR_FEDUWhlTqReqSmoothDelay_Nm] -> VTQR_SNOWFEDURateLimitInc_Nm/3
  [VINP_FrPTCSActive_flg] -> Logical Operator2/1
  If1/3 -> VTQR_ESCAPEFEDURateLimitInc_Nm/Action
  Equal5/1 -> If1/6
  [VINP_FrntAxlTrqReqDrv_Nm] -> Relational Operator8/2
  Logical Operator2/1 -> If1/2
  VTQR_NORMALFEDURateLimitInc_Nm/1 -> [VTQR_NORMALFEDURateLimitInc_Nm]  "VTQR_NORMALFEDURateLimitInc_Nm"
  Equal3/1 -> Logical Operator2/2
  [VINP_IVISnowModeCmd_flg] -> If1/4
  [VDHP_ActAPSPosn_pct] -> VTQR_SPORTFEDURateLimitInc_Nm/1
  [VTQD_FrShaftSpd_rpm] -> VTQR_ESCAPEFEDURateLimitInc_Nm/2
  If1/4 -> VTQR_SNOWFEDURateLimitInc_Nm/Action
  [VTQD_TqTargetShaftSpd_rpm] -> VTQR_NORMALFEDURateLimitInc_Nm/2
  [VTQD_CoordWhlTqDemFr_Nm] -> Relational Operator8/1
  VTQR_TCSFEDURateLimitInc_Nm/1 -> [VTQR_TCSFEDURateLimitInc_Nm]  "VTQR_TCSFEDURateLimitInc_Nm"
  VTQR_LHMFEDURateLimitInc_Nm/1 -> [VTQR_LHMFEDURateLimitInc_Nm]  "VTQR_LHMFEDURateLimitInc_Nm"
  If1/2 -> VTQR_TCSFEDURateLimitInc_Nm/Action
  [VDHP_ActAPSPosn_pct] -> VTQR_ESCAPEFEDURateLimitInc_Nm/1
  Constant/1 -> Equal3/2
  If1/1 -> VTQR_LHMFEDURateLimitInc_Nm/Action
  If1/6 -> VTQR_ECOFEDURateLimitInc_Nm/Action
  [VTQD_TqTargetShaftSpd_rpm] -> VTQR_ECOFEDURateLimitInc_Nm/2
  [VDHP_ActAPSPosn_pct] -> VTQR_SNOWFEDURateLimitInc_Nm/1
  If1/5 -> VTQR_NORMALFEDURateLimitInc_Nm/Action
  If1/7 -> VTQR_SPORTFEDURateLimitInc_Nm/Action
  [VTQD_IVIRockModeEn_flg] -> If1/3
  [VTQR_FEDUWhlTqReqSmoothDelay_Nm] -> VTQR_ECOFEDURateLimitInc_Nm/4
  [VDHP_ActAPSPosn_pct] -> VTQR_TCSFEDURateLimitInc_Nm/1
  VTQR_SNOWFEDURateLimitInc_Nm/1 -> [VTQR_SNOWFEDURateLimitInc_Nm]  "VTQR_SNOWFEDURateLimitInc_Nm"
  [VTQD_TqTargetShaftSpd_rpm] -> VTQR_TCSFEDURateLimitInc_Nm/2
  [VDHP_ActAPSPosn_pct] -> VTQR_NORMALFEDURateLimitInc_Nm/1
  Equal6/1 -> If1/5
  [VTQD_LimpHomeAct_flg] -> Logical Operator4/1
  [VTQD_TqTargetShaftSpd_rpm] -> VTQR_SNOWFEDURateLimitInc_Nm/2
  [VTQR_FEDUWhlTqReqSmoothDelay_Nm] -> VTQR_SPORTFEDURateLimitInc_Nm/4
  [VTQD_RegenMode_enum] -> VTQR_SPORTFEDURateLimitInc_Nm/3
  [VTQR_FEDUWhlTqReqSmoothDelay_Nm] -> VTQR_NORMALFEDURateLimitInc_Nm/4
  VTQR_SPORTFEDURateLimitInc_Nm/1 -> [VTQR_SPORTFEDURateLimitInc_Nm]  "VTQR_SPORTFEDURateLimitInc_Nm"
  [VTQD_RegenMode_enum] -> VTQR_ECOFEDURateLimitInc_Nm/3
  [VTQR_EVDriveMode_enum] -> Equal5/1
  Equal8/1 -> If1/7
  Logical Operator5/1 -> Logical Operator4/2
  [VTQD_RegenMode_enum] -> VTQR_NORMALFEDURateLimitInc_Nm/3
  [VTQR_EVDriveMode_enum] -> Equal6/1
  Constant9/1 -> Equal8/2
  Constant8/1 -> Equal6/2
  Relational Operator8/1 -> Logical Operator2/3
  [VDHP_ActAPSPosn_pct] -> VTQR_LHMFEDURateLimitInc_Nm/1
  [VTQD_TqTargetShaftSpd_rpm] -> VTQR_SPORTFEDURateLimitInc_Nm/2
  VTQR_ESCAPEFEDURateLimitInc_Nm/1 -> [VTQR_ESCAPEFEDURateLimitInc_Nm]  "VTQR_ESCAPEFEDURateLimitInc_Nm"
  [VINP_VehicleType_enum] -> Equal3/1
  [VTQD_EVDriveModeValid_flg] -> Logical Operator5/1
  [VDHP_ActAPSPosn_pct] -> VTQR_ECOFEDURateLimitInc_Nm/1
  Logical Operator4/1 -> If1/1
  Constant7/1 -> Equal5/2
  [VTQD_TqTargetShaftSpd_rpm] -> VTQR_LHMFEDURateLimitInc_Nm/2
  VTQR_ECOFEDURateLimitInc_Nm/1 -> [VTQR_ECOFEDURateLimitInc_Nm]  "VTQR_ECOFEDURateLimitInc_Nm"
  [VTQD_RegenMode_enum] -> VTQR_ECOFEDURateLimitDec_Nm/3
  [VTQR_FEDUWhlTqReqSmoothDelay_Nm] -> VTQR_TCSFEDURateLimitDec_Nm/1
  If2/4 -> VTQR_SNOWFEDURateLimitDec_Nm/Action
  [VTQD_CoordWhlTqDemFr_Nm] -> Relational Operator9/1
  Logical Operator3/1 -> If2/2
  [VINP_VehicleType_enum] -> Equal4/1
  [VTQD_FrShaftSpd_rpm] -> VTQR_ESCAPEFEDURateLimitDec_Nm/2
  If2/2 -> VTQR_TCSFEDURateLimitDec_Nm/Action
  VTQR_TCSFEDURateLimitDec_Nm/1 -> [VTQR_TCSFEDURateLimitDec_Nm]  "VTQR_TCSFEDURateLimitDec_Nm"
  If2/5 -> VTQR_NORMALFEDURateLimitDec_Nm/Action
  If2/1 -> VTQR_LHMFEDURateLimitDec_Nm/Action
  [VINP_FrPTCSActive_flg] -> Logical Operator3/1
  [VTQD_TqTargetShaftSpd_rpm] -> VTQR_SNOWFEDURateLimitDec_Nm/2
  [VTQD_IVIRockModeEn_flg] -> If2/3
  [VTQD_LimpHomeAct_flg] -> Logical Operator6/1
  VTQR_SNOWFEDURateLimitDec_Nm/1 -> [VTQR_SNOWFEDURateLimitDec_Nm]  "VTQR_SNOWFEDURateLimitDec_Nm"
  VTQR_NORMALFEDURateLimitDec_Nm/1 -> [VTQR_NORMALFEDURateLimitDec_Nm]  "VTQR_NORMALFEDURateLimitDec_Nm"
  [VTQR_FEDUWhlTqReqSmoothDelay_Nm] -> VTQR_SNOWFEDURateLimitDec_Nm/1
  [VTQD_EVDriveModeValid_flg] -> Logical Operator1/1
  If2/3 -> VTQR_ESCAPEFEDURateLimitDec_Nm/Action
  VTQR_LHMFEDURateLimitDec_Nm/1 -> [VTQR_LHMFEDURateLimitDec_Nm]  "VTQR_LHMFEDURateLimitDec_Nm"
  VTQR_ESCAPEFEDURateLimitDec_Nm/1 -> [VTQR_ESCAPEFEDURateLimitDec_Nm]  "VTQR_ESCAPEFEDURateLimitDec_Nm"
  Equal13/1 -> If2/5
  [VTQR_FEDUWhlTqReqSmoothDelay_Nm] -> VTQR_ESCAPEFEDURateLimitDec_Nm/1
  Equal12/1 -> If2/6
  [VINP_IVISnowModeCmd_flg] -> If2/4
  If2/6 -> VTQR_ECOFEDURateLimitDec_Nm/Action
  [VTQD_TqTargetShaftSpd_rpm] -> VTQR_TCSFEDURateLimitDec_Nm/2
  [VTQR_FEDUWhlTqReqSmoothDelay_Nm] -> VTQR_LHMFEDURateLimitDec_Nm/1
  [VINP_FrntAxlTrqReqDrv_Nm] -> Relational Operator9/2
  [VTQD_TqTargetShaftSpd_rpm] -> VTQR_LHMFEDURateLimitDec_Nm/2
  [VTQD_TqTargetShaftSpd_rpm] -> VTQR_SPORTFEDURateLimitDec_Nm/2
  [VTQD_TqTargetShaftSpd_rpm] -> VTQR_NORMALFEDURateLimitDec_Nm/2
  [VTQR_FEDUWhlTqReqSmoothDelay_Nm] -> VTQR_NORMALFEDURateLimitDec_Nm/1
  Relational Operator9/1 -> Logical Operator3/3
  Constant15/1 -> Equal13/2
  [VTQR_EVDriveMode_enum] -> Equal13/1
  [VTQR_EVDriveMode_enum] -> Equal12/1
  Logical Operator1/1 -> Logical Operator6/2
  VTQR_ECOFEDURateLimitDec_Nm/1 -> [VTQR_ECOFEDURateLimitDec_Nm]  "VTQR_ECOFEDURateLimitDec_Nm"
  [VTQR_FEDUWhlTqReqSmoothDelay_Nm] -> VTQR_SPORTFEDURateLimitDec_Nm/1
  [VTQD_RegenMode_enum] -> VTQR_SPORTFEDURateLimitDec_Nm/3
  [VTQD_RegenMode_enum] -> VTQR_NORMALFEDURateLimitDec_Nm/3
  Equal15/1 -> If2/7
  Logical Operator6/1 -> If2/1
  Constant14/1 -> Equal12/2
  Constant17/1 -> Equal15/2
  VTQR_SPORTFEDURateLimitDec_Nm/1 -> [VTQR_SPORTFEDURateLimitDec_Nm]  "VTQR_SPORTFEDURateLimitDec_Nm"
  [VTQR_EVDriveMode_enum] -> Equal15/1
  If2/7 -> VTQR_SPORTFEDURateLimitDec_Nm/Action
  [VTQD_TqTargetShaftSpd_rpm] -> VTQR_ECOFEDURateLimitDec_Nm/2
  [VTQR_FEDUWhlTqReqSmoothDelay_Nm] -> VTQR_ECOFEDURateLimitDec_Nm/1
  Constant22/1 -> Equal4/2
  Equal4/1 -> Logical Operator3/2
  [VTQR_TCSFEDURateLimitInc_Nm] -> Merge1/2
  [VTQR_LHMFEDURateLimitInc_Nm] -> Merge1/1
  [VTQR_NORMALFEDURateLimitInc_Nm] -> Merge1/5
  [VTQR_SNOWFEDURateLimitInc_Nm] -> Merge1/4
  [VTQR_ESCAPEFEDURateLimitInc_Nm] -> Merge1/3
  [VTQR_SPORTFEDURateLimitInc_Nm] -> Merge1/7
  [VTQR_ECOFEDURateLimitInc_Nm] -> Merge1/6
  Delay/1 -> Switch4/1
  [VTQR_EVDriveMode_enum] -> Detect Change/1
  Detect Change/1 -> SR_Latch1/1
  Switch4/1 -> [VTQR_FEDURateLimitInc_Nm], Delay/1  "VTQR_FEDURateLimitInc_Nm"
  [VTQR_FrDrModChangeReset_flg] -> SR_Latch1/2
  SR_Latch1/1 -> Switch4/2, [VTQR_FrDrModIncLatch_flg]
  Merge1/1 -> Switch4/3
  Switch5/1 -> [VTQR_FEDURateLimitDec_Nm], Delay2/1  "VTQR_FEDURateLimitDec_Nm"
  [VTQR_LHMFEDURateLimitDec_Nm] -> Merge2/1
  [VTQR_TCSFEDURateLimitDec_Nm] -> Merge2/2
  [VTQR_ESCAPEFEDURateLimitDec_Nm] -> Merge2/3
  [VTQR_SNOWFEDURateLimitDec_Nm] -> Merge2/4
  [VTQR_SPORTFEDURateLimitDec_Nm] -> Merge2/7
  [VTQR_NORMALFEDURateLimitDec_Nm] -> Merge2/5
  [VTQR_ECOFEDURateLimitDec_Nm] -> Merge2/6
  [VTQR_EVDriveMode_enum] -> Detect Change1/1
  Detect Change1/1 -> SR_Latch2/1
  [VTQR_FrDrModChangeReset_flg] -> SR_Latch2/2
  SR_Latch2/1 -> Switch5/2, [VTQR_FrDrModDecLatch_flg]
  Merge2/1 -> Switch5/3
  Delay2/1 -> Switch5/1
  Add1/1 -> Abs4/1
  Abs/1 -> Relational Operator5/1
  [VTQR_FrDrModDecLatch_flg] -> Delay4/1
  [VTQR_FrFirstOrderInpTq_Nm] -> Add/2
  OR2/1 -> [VTQR_FrDrModChangeReset_flg]  "VTQR_FrDrModChangeReset_flg"
  Abs4/1 -> Relational Operator6/1
  Delay3/1 -> OR3/1
  OR3/1 -> AND4/2
  Delay1/1 -> Add1/1
  [VTQR_FrFirstOrderInpTq_Nm] -> Delay1/1
  Constant5/1 -> Relational Operator5/2
  Add/1 -> Abs/1
  Constant11/1 -> Relational Operator6/2
  [VTQR_FrDrModIncLatch_flg] -> Delay3/1
  Relational Operator5/1 -> OR2/1
  Relational Operator6/1 -> AND4/1
  Delay4/1 -> OR3/2
  [VTQR_NoABSFEDUWhlTqReq_Nm] -> Add/1
  AND4/1 -> OR2/2
  [VTQR_FrFirstOrderInpTq_Nm] -> Add1/2
  [VTQR_FEDURateLimitDec_Nm] -> Mux/2
  [VTQR_FEDURateLimitInc_Nm] -> Mux/1
  Mux/1 -> [VTQR_DriveModeTqIncDec_Nm]
  If3/4 -> VTQR_VMCFEDUIncDec_Nm/Action
  If3/5 -> Drive mode/Action
  [VTQR_DriveModeTqIncDec_Nm] -> Drive mode/1(VTQR_DriveModeTqIncDec_Nm)
  Drive mode/1(VTQR_OutDriveModeTqIncDec_Nm) -> [VTQR_OutDriveModeTqIncDec_Nm]  "VTQR_OutDriveModeTqIncDec_Nm"
  [VTQR_OutDriveModeTqIncDec_Nm] -> Merge/5
  VVMC_EstSlope_Deg/1 -> [VVMC_EstSlope_Deg]
  [VVMC_EstSlope_Deg] -> VTQR_CreepFEDUTqIncDecSR_Nm/3(VVMC_EstSlope_Deg)
